simulink model "multibus_test"  (R2018a)
settings: Solver=VariableStepAuto  StartTime=0.0  StopTime=10.0  RelTol=1e-3
model workspace (MAT data in the model file):
  Sig = Simulink.Signal
  Sig.DataType = 'x2'
  Sig.Dimensions = -1
  Sig.DimensionsMode = 'auto'
  Sig.Complexity = 'auto'
  Sig.SampleTime = -1
  Sig.SamplingMode = 'auto'
  x1 = Simulink.Signal
  x1.DataType = 'auto'
  x1.Dimensions = -1
  x1.DimensionsMode = 'auto'
  x1.Complexity = 'auto'
  x1.SampleTime = -1
  x1.SamplingMode = 'auto'
settings Model: DataDictionary=test_dd.sldd  Creator=Michael Girbino  LastModifiedBy=Michael Girbino
settings DebuggingCC: BusObjectLabelMismatch=none

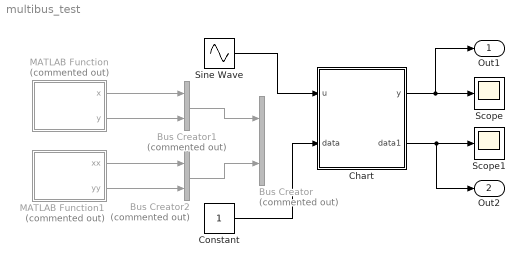
== system multibus_test ==
  Bus Creator : BusCreator  Commented=on  Inputs=2  OutDataTypeStr=Bus: in_busc
  Bus Creator1 : BusCreator  Commented=on  Inputs=2  OutDataTypeStr=Bus: in_busa
  Bus Creator2 : BusCreator  Commented=on  Inputs=2  OutDataTypeStr=Bus: in_busb
  Chart : Stateflow chart  TreatAsAtomicUnit=on
  Constant : Constant
  MATLAB Function : MATLAB Function  Commented=on  TreatAsAtomicUnit=on
  MATLAB Function1 : MATLAB Function  Commented=on  TreatAsAtomicUnit=on
  Scope : Scope
  Scope1 : Scope
  Sine Wave : Sin  SampleTime=0
  Out1 : Outport  SignalName=x1  InitialOutput=0
  Out2 : Outport  Port=2  SignalName=x2  InitialOutput=0
  wires:
  Sine Wave/1 -> Chart/1(u)
  Chart/1(y) -> Out1/1, Scope/1
  Chart/2(data1) -> Out2/1, Scope1/1
  Bus Creator2/1 -> Bus Creator/2
  Bus Creator1/1 -> Bus Creator/1
  MATLAB Function/1(x) -> Bus Creator1/1
  MATLAB Function/2(y) -> Bus Creator1/2
  MATLAB Function1/1(xx) -> Bus Creator2/1
  MATLAB Function1/2(yy) -> Bus Creator2/2
  Constant/1 -> Chart/2(data)

== matlab function multibus_test/MATLAB Function1 ==
  data: xx output; yy output
function [xx,yy] = in_numeric
    xx = 1.234;
    yy = 2.3456;
end

== matlab function multibus_test/MATLAB Function ==
  data: x output; y output
function [x,y] = in_tf
    x = true;
    y = false;
end

== stateflow chart multibus_test/Chart ==
  state State1 %State Name
    entry: y = -1; % entry action
    entry: data1 = data;%spaghetti(data);
    % during:
  state State2
    entry: y = 1;
    entry: data1 = data * 2; % 0;
  (default) -> State1 %State Name
  State1 %State Name -> State2 : [u <= 0]
      | % [transition condition]{action}
  State2 -> State1 %State Name : [u > 0]
  data: inp function_input; outp function_output; u input; y output; data input size=1; data1 output
  function outp = spaghetti(inp):
    | function outp = spaghetti(inp)
    |     outp = inp.x;
    | end
